simulink model "task2b"  (R2018b)
settings: Solver=VariableStepAuto  StartTime=0.0  StopTime=10.0  RelTol=1e-3
settings Model: Creator=root  LastModifiedBy=root

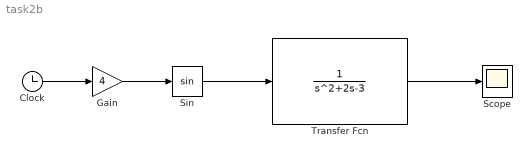
== system task2b ==
  Clock : Clock
  Gain : Gain  Gain=4
  Scope : Scope
  Sin : Trigonometry
  Transfer Fcn : TransferFcn  Denominator=[1 2 -3]
  wires:
  Clock/1 -> Gain/1
  Gain/1 -> Sin/1
  Sin/1 -> Transfer Fcn/1
  Transfer Fcn/1 -> Scope/1
